simulink library "xblocks_library_pfbs"  (Simulink 7.6)
settings: Solver=ode45  SolverMode=SingleTasking  StartTime=0.0  StopTime=10.0  RelTol=1e-3
libraries: xbsIndex_r4 x369, monroe_library x47
(part 2 of 7)

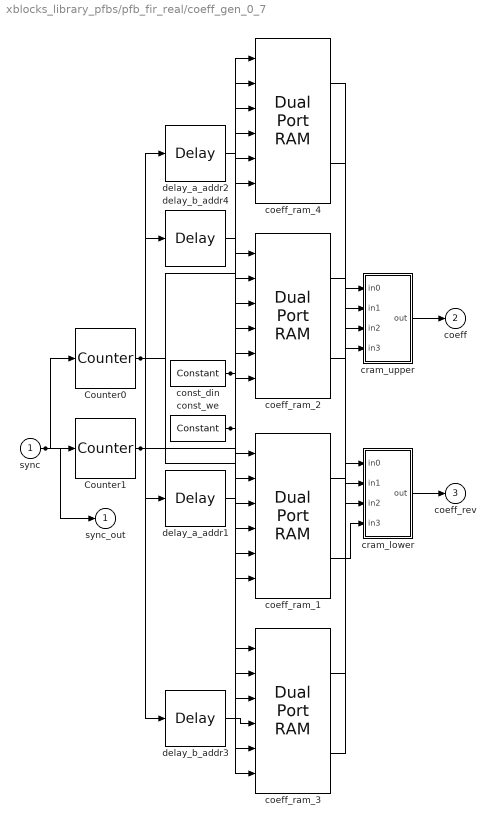
== system xblocks_library_pfbs/pfb_fir_real/coeff_gen_0_7 ==
  sync : Inport
  Counter0 : xbsIndex_r4/Counter  cnt_type=Free Running  cnt_to=Inf  operation=Up  start_count=8  cnt_by_val=1  arith_type=Unsigned  n_bits=11  bin_pt=0  load_pin=off  rst=on  en=off  explicit_period=on  period=1  dbl_ovrd=off  use_behavioral_HDL=off  implementation=Fabric  block_type=counter
  Counter1 : xbsIndex_r4/Counter  cnt_type=Free Running  cnt_to=Inf  operation=Down  start_count=2039  cnt_by_val=1  arith_type=Unsigned  n_bits=11  bin_pt=0  load_pin=off  rst=on  en=off  explicit_period=on  period=1  dbl_ovrd=off  use_behavioral_HDL=off  implementation=Fabric  block_type=counter
  coeff_ram_1 : xbsIndex_r4/Dual Port RAM  depth=2048  initVector=[-1.22072174986674e-006 -2.07573634838521e-005 -4.03037029782619e-005 -5.98598996980381e-005 -7.94261132606548e-005 -9.90025034347064e-005 -0.000118589230138382 -0.00013818645343805 -0.000157794333546782 -0.000177413030822893 -0.000197042705768457 -0.000216683519027889 -0.000236335631386401 -0.00025599920376858 -0.000275674397236896 -0.000295361372990216 -0.000315060292362373 -0.00033477131682061 -0.000354494607964151 -0.000374230327522695 -0.000393978637354936 -0.000413739699447062 -0.000433513675911303 -0.000453300728984377 -0.000473101021026037 -0.000492914714517562 -0.000512741972060248 -0.000532582956373951 -0.00055243783029552 -0.000572306756777332 -0.000592189898885775 -0.000612087419799743 -0.000631999482809111 -0.00065192625131327 -0.000671867888819539 -0.000691824558941702 -0.000711796425398473 -0.000731783652011965 -0.000751786402706218 -0.0007718048415056 -0.000791839132533333 -0.000811889440009951 -0.00083195592825177 -0.000852038761669347 -0.000872138104765997 -0.000892254122136178 -0.000912386978464012 -0.000932536838521728 -0.000952703867168116 -0.000972888229347025 -0.000993090090085754 -0.00101330961449355 -0.00103354696776005 -0.00105380231515375 -0.00107407582202039 -0.00109436765378152 -0.00111467797593281 -0.0011350069540426 -0.00115535475375027 -0.00117572154076472 -0.00119610748086284 -0.00121651273988784 -0.00123693748374781 -0.00125738187841406 -0.00127784608991962 -0.0012983302843576 -0.0013188346278797 -0.00133935928669459 -0.00135990442706632 -0.00138047021531278 -0.00140105681780409 -0.00142166440096108 -0.00144229313125365 -0.00146294317519918 -0.001483614699361 -0.00150430787034677 -0.0015250228548069 -0.00154575981943296 -0.00156651893095611 -0.00158730035614545 -0.00160810426180649 -0.00162893081477952 -0.00164978018193805 -0.00167065253018717 -0.00169154802646197 -0.00171246683772591 -0.00173340913096929 -0.00175437507320756 -0.00177536483147979 -0.00179637857284702 -0.00181741646439064 -0.00183847867321083 -0.00185956536642487 -0.00188067671116564 -0.00190181287457992 -0.00192297402382678 -0.001944160326076 -0.00196537194850642 -0.00198660905830434 -0.00200787182266191 -0.00202916040877547 -0.00205047498384395 -0.00207181571506724 -0.00209318276964456 -0.00211457631477287 -0.00213599651764518 -0.00215744354544895 -0.00217891756536446 -0.00220041874456319 -0.00222194725020613 -0.00224350324944225 -0.00226508690940674 -0.00228669839721945 -0.00230833787998322 -0.00233000552478227 -0.00235170149868053 -0.00237342596871999 -0.0023951791019191 -0.00241696106527107 -0.00243877202574225 -0.00246061215027048 -0.00248248160576349 -0.00250438055909712 -0.00252630917711381 -0.00254826762662086 -0.0025702560743888 -0.00259227468714977 -0.00261432363159582 -0.00263640307437723 -0.00265851318210093 -0.00268065412132879 -0.00270282605857593 -0.00272502916030915 -0.0027472635929452 -0.00276952952284908 -0.00279182711633249 -0.00281415653965204 -0.0028365179590077 -0.00285891154054103 -0.00288133745033356 -0.00290379585440513 -0.00292628691871219 -0.00294881080914613 -0.00297136769153166 -0.00299395773162504 -0.0030165810951125 -0.00303923794760849 -0.00306192845465405 -0.00308465278171512 -0.00310741109418087 -0.00313020355736198 -0.003153030336489 -0.00317589159671066 -0.00319878750309216 -0.00322171822061356 -0.00324468391416799 -0.00326768474856006 -0.0032907208885041 -0.00331379249862253 -0.00333689974344414 -0.00336004278740241 -0.00338322179483382 -0.00340643692997616 -0.00342968835696683 -0.00345297623984116 -0.00347630074253073 -0.00349966202886164 -0.00352306026255283 -0.00354649560721441 -0.00356996822634591 -0.00359347828333467 -0.00361702594145403 -0.00364061136386173 -0.00366423471359816 -0.00368789615358466 -0.00371159584662182 -0.00373533395538786 -0.00375911064243679 -0.00378292607019678 -0.00380678040096848 -0.00383067379692324 -0.00385460642010154 -0.00387857843241112 -0.00390258999562537 -0.00392664127138162 -0.00395073242117942 -0.00397486360637879 -0.00399903498819863 ...(+37251 chars)]  distributed_mem=Block RAM  init_a=0  init_b=0  rst_a=off  rst_b=off  en_a=off  en_b=off  latency=2  write_mode_A=No Read On Write  write_mode_B=No Read On Write  dbl_ovrd=off  optimize=Area  use_rpm=on  block_type=dpram
  coeff_ram_2 : xbsIndex_r4/Dual Port RAM  depth=2048  initVector=[1.64803315783465e-005 0.000280485521810809 0.000545093027402636 0.00081030310745065 0.00107611601953105 0.00134253201969671 0.00160955136247522 0.00187717430086683 0.00214540108634176 0.00241423196883855 0.00268366719676137 0.00295370701697797 0.00322435167481777 0.00349560141406919 0.00376745647697767 0.00403991710424374 0.00431298353502034 0.00458665600691093 0.00486093475596747 0.00513582001668779 0.00541131202201398 0.00568741100332972 0.00596411719045836 0.00624143081166097 0.00651935209363378 0.0067978812615062 0.00707701853883898 0.00735676414762159 0.00763711830827029 0.00791808123962629 0.00819965315895307 0.00848183428193485 0.008764624822674 0.00904802499368911 0.00933203500591316 0.00961665506869093 0.00990188538977718 0.0101877261753347 0.010474177629932 0.010761239956541 0.0110489133565358 0.0113371980296895 0.0116260941741733 0.0119156019865533 0.0122057216617891 0.012496453393232 0.0127877973726222 0.0130797537900872 0.0133723228341399 0.0136655046916763 0.0139592995479734 0.0142537075866877 0.0145487289898524 0.0148443639378762 0.0151406126095406 0.0154374751819983 0.0157349518307712 0.0160330427297483 0.0163317480511835 0.0166310679656943 0.0169310026422588 0.0172315522482147 0.017532716949257 0.0178344969094354 0.0181368922911536 0.0184399032551663 0.0187435299605775 0.019047772564839 0.0193526312237478 0.0196581060914447 0.0199641973204122 0.0202709050614723 0.020578229463785 0.0208861706748463 0.021194728840486 0.0215039041048662 0.0218136966104791 0.0221241064981451 0.0224351339070113 0.0227467789745491 0.0230590418365527 0.0233719226271371 0.0236854214787361 0.0239995385221007 0.0243142738862971 0.0246296276987047 0.0249456000850147 0.0252621911692277 0.0255794010736522 0.0258972299189029 0.0262156778238985 0.0265347449058598 0.0268544312803088 0.0271747370610656 0.0274956623602476 0.0278172072882672 0.02813937195383 0.0284621564639336 0.0287855609238648 0.0291095854371986 0.0294342301057965 0.029759495029804 0.0300853803076495 0.0304118860360423 0.0307390123099709 0.0310667592227011 0.0313951268657746 0.0317241153290068 0.0320537247004856 0.0323839550665691 0.0327148065118842 0.0330462791193253 0.0333783729700515 0.0337110881434859 0.0340444247173137 0.03437838276748 0.0347129623681887 0.0350481635919005 0.0353839865093313 0.0357204311894507 0.0360574976994799 0.0363951861048906 0.0367334964694028 0.0370724288549838 0.0374119833218455 0.0377521599284443 0.0380929587314779 0.0384343797858845 0.0387764231448415 0.0391190888597629 0.0394623769802986 0.0398062875543322 0.0401508206279795 0.0404959762455876 0.0408417544497322 0.0411881552812166 0.0415351787790705 0.0418828249805475 0.0422310939211244 0.0425799856344993 0.0429295001525897 0.0432796375055317 0.0436303977216779 0.0439817808275958 0.0443337868480668 0.0446864158060843 0.045039667722852 0.0453935426177829 0.0457480405084974 0.0461031614108218 0.0464589053387873 0.0468152723046275 0.0471722623187784 0.0475298753898752 0.0478881115247521 0.0482469707284406 0.0486064530041675 0.0489665583533539 0.0493272867756139 0.0496886382687526 0.0500506128287651 0.0504132104498352 0.0507764311243331 0.0511402748428151 0.0515047415940217 0.0518698313648757 0.0522355441404818 0.0526018799041244 0.0529688386372664 0.0533364203195482 0.0537046249287857 0.0540734524409694 0.0544429028302629 0.0548129760690015 0.0551836721276905 0.0555549909750048 0.0559269325777866 0.0562994969010446 0.0566726839079523 0.0570464935598469 0.0574209258162282 0.0577959806347566 0.0581716579712526 0.058547957779695 0.0589248800122198 0.0593024246191185 0.0596805915488377 0.0600593807479768 0.0604387921612875 0.0608188257316721 0.0611994814001824 0.0615807591060186 0.0619626587865276 0.062345180377202 0.0627283238116794 0.0631120890217402 0.063496475937307 0.0638814844864433 0.064267114595352 0.0646533661883749 0.0650402391879906 0.0654277335148137 0.065815849087594 0.0662045858232146 0.0665939436366913 0.0669839224411714 0.067374522147932 0.0677657426663793 0.0681575839040475 ...(+32994 chars)]  distributed_mem=Block RAM  init_a=0  init_b=0  rst_a=off  rst_b=off  en_a=off  en_b=off  latency=2  write_mode_A=No Read On Write  write_mode_B=No Read On Write  dbl_ovrd=off  optimize=Area  use_rpm=on  block_type=dpram
  coeff_ram_3 : xbsIndex_r4/Dual Port RAM  depth=2048  initVector=[0.999999997939492 0.999999404513317 0.999997756108682 0.999995052729556 0.999991294382447 0.999986481076405 0.99998061282302 0.999973689636421 0.999965711533277 0.999956678532798 0.999946590656734 0.999935447929374 0.999923250377545 0.999909998030619 0.999895690920501 0.999880329081641 0.999863912551025 0.999846441368179 0.999827915575169 0.9998083352166 0.999787700339613 0.999766010993892 0.999743267231656 0.999719469107664 0.999694616679213 0.999668710006138 0.999641749150811 0.999613734178142 0.999584665155579 0.999554542153107 0.999523365243246 0.999491134501054 0.999457850004128 0.999423511832596 0.999388120069126 0.999351674798921 0.999314176109716 0.999275624091786 0.999236018837938 0.999195360443513 0.999153649006388 0.999110884626972 0.999067067408209 0.999022197455575 0.99897627487708 0.998929299783265 0.998881272287205 0.998832192504505 0.998782060553301 0.998730876554262 0.998678640630587 0.998625352908004 0.998571013514771 0.998515622581677 0.998459180242038 0.998401686631699 0.998343141889033 0.998283546154941 0.998222899572851 0.998161202288718 0.998098454451022 0.998034656210769 0.997969807721491 0.997903909139244 0.997836960622608 0.997768962332688 0.997699914433111 0.997629817090025 0.997558670472104 0.99748647475054 0.997413230099047 0.997338936693861 0.997263594713734 0.997187204339941 0.997109765756274 0.997031279149043 0.996951744707075 0.996871162621715 0.996789533086822 0.996706856298774 0.99662313245646 0.996538361761285 0.996452544417169 0.996365680630542 0.996277770610348 0.996188814568043 0.996098812717592 0.996007765275471 0.995915672460666 0.995822534494672 0.99572835160149 0.99563312400763 0.995536851942108 0.995439535636445 0.995341175324669 0.99524177124331 0.995141323631404 0.995039832730486 0.994937298784596 0.994833722040274 0.994729102746561 0.994623441154996 0.994516737519617 0.994408992096962 0.994300205146064 0.99419037692845 0.994079507708148 0.993967597751674 0.993854647328043 0.993740656708758 0.993625626167818 0.99350955598171 0.993392446429412 0.99327429779239 0.993155110354601 0.993034884402484 0.99291362022497 0.992791318113473 0.992667978361889 0.9925436012666 0.992418187126472 0.992291736242848 0.992164248919555 0.992035725462898 0.99190616618166 0.991775571387104 0.991643941392966 0.99151127651546 0.991377577073273 0.991242843387566 0.991107075781971 0.990970274582594 0.990832440118009 0.990693572719259 0.990553672719856 0.990412740455777 0.990270776265469 0.990127780489838 0.989983753472259 0.989838695558565 0.989692607097053 0.989545488438481 0.989397339936062 0.989248161945471 0.989097954824838 0.988946718934749 0.988794454638243 0.988641162300815 0.988486842290409 0.988331494977421 0.988175120734697 0.988017719937532 0.987859292963666 0.987699840193286 0.987539362009025 0.987377858795956 0.987215330941599 0.98705177883591 0.986887202871287 0.986721603442567 0.986554980947023 0.986387335784363 0.986218668356731 0.986048979068703 0.985878268327288 0.985706536541923 0.985533784124477 0.985360011489246 0.985185219052951 0.985009407234739 0.98483257645618 0.984654727141269 0.984475859716419 0.984295974610463 0.984115072254653 0.983933153082657 0.983750217530559 0.983566266036857 0.98338129904246 0.983195316990689 0.983008320327275 0.982820309500356 0.982631284960478 0.982441247160591 0.98225019655605 0.98205813360461 0.981865058766429 0.981670972504062 0.981475875282465 0.981279767568986 0.981082649833371 0.980884522547757 0.980685386186674 0.980485241227041 0.980284088148167 0.980081927431746 0.979878759561857 0.979674585024966 0.979469404309918 0.97926321790794 0.979056026312637 0.978847830019992 0.978638629528364 0.978428425338485 0.978217217953461 0.978005007878768 0.977791795622251 0.977577581694123 0.977362366606961 0.97714615087571 0.976928935017675 0.97671071955252 0.976491505002273 0.976271291891314 0.976050080746383 0.975827872096571 0.975604666473324 0.975380464410436 0.975155266444051 0.974929073112661 0.9747018849571 0.97447370252055 0.974244526348531 ...(+32991 chars)]  distributed_mem=Block RAM  init_a=0  init_b=0  rst_a=off  rst_b=off  en_a=off  en_b=off  latency=2  write_mode_A=No Read On Write  write_mode_B=No Read On Write  dbl_ovrd=off  optimize=Area  use_rpm=on  block_type=dpram
  coeff_ram_4 : xbsIndex_r4/Dual Port RAM  depth=2048  initVector=[-1.64779798652932e-005 -0.000279805876911002 -0.000542532014217755 -0.000804656655620616 -0.00106618006646648 -0.00132710251361138 -0.00158742426541843 -0.00184714559175581 -0.00210626676399397 -0.00236478805500397 -0.00262270973915464 -0.0028800320923106 -0.00313675539183012 -0.00339287991656244 -0.00364840594684571 -0.00390333376450485 -0.00415766365284889 -0.00441139589666884 -0.0046645307822356 -0.00491706859729718 -0.0051690096310769 -0.00542035417427064 -0.00567110251904467 -0.00592125495903356 -0.00617081178933743 -0.00641977330651982 -0.00666813980860556 -0.006915911595078 -0.00716308896687689 -0.00740967222639621 -0.00765566167748135 -0.0079010576254273 -0.00814586037697581 -0.0083900702403132 -0.00863368752506823 -0.00887671254230929 -0.00911914560454224 -0.00936098702570823 -0.00960223712118088 -0.00984289620776415 -0.0100829646036901 -0.0103224426286159 -0.0105613306036224 -0.0107996288512106 -0.0110373376953001 -0.0112744574612263 -0.0115109884757381 -0.0117469310669953 -0.0119822855645665 -0.0122170522994264 -0.0124512316039533 -0.0126848238119272 -0.0129178292585265 -0.0131502482803265 -0.013382081215296 -0.0136133284027958 -0.0138439901835755 -0.0140740668997713 -0.0143035588949036 -0.0145324665138748 -0.014760790102966 -0.0149885300098353 -0.0152156865835152 -0.0154422601744097 -0.0156682511342925 -0.0158936598163037 -0.0161184865749479 -0.0163427317660917 -0.0165663957469608 -0.0167894788761377 -0.0170119815135596 -0.0172339040205152 -0.0174552467596424 -0.0176760100949264 -0.017896194391696 -0.0181158000166224 -0.0183348273377156 -0.0185532767243224 -0.0187711485471239 -0.0189884431781327 -0.0192051609906904 -0.0194213023594655 -0.0196368676604501 -0.0198518572709579 -0.0200662715696215 -0.02028011093639 -0.0204933757525261 -0.0207060664006037 -0.0209181832645053 -0.0211297267294199 -0.0213406971818396 -0.0215510950095574 -0.021760920601665 -0.0219701743485495 -0.0221788566418916 -0.0223869678746622 -0.0225945084411204 -0.0228014787368109 -0.0230078791585608 -0.0232137101044777 -0.0234189719739467 -0.0236236651676281 -0.0238277900874542 -0.0240313471366275 -0.0242343367196175 -0.024436759242158 -0.0246386151112452 -0.0248399047351341 -0.0250406285233368 -0.0252407868866192 -0.0254403802369984 -0.0256394089877407 -0.0258378735533583 -0.0260357743496066 -0.0262331117934824 -0.0264298863032203 -0.0266260982982904 -0.0268217481993957 -0.0270168364284696 -0.0272113634086729 -0.0274053295643913 -0.0275987353212325 -0.0277915811060242 -0.0279838673468106 -0.0281755944728502 -0.028366762914613 -0.0285573731037779 -0.0287474254732299 -0.0289369204570574 -0.0291258584905497 -0.0293142400101941 -0.0295020654536733 -0.0296893352598626 -0.0298760498688275 -0.0300622097218205 -0.0302478152612788 -0.0304328669308217 -0.0306173651752471 -0.0308013104405299 -0.0309847031738184 -0.0311675438234319 -0.0313498328388582 -0.0315315706707505 -0.0317127577709246 -0.0318933945923569 -0.0320734815891808 -0.0322530192166844 -0.0324320079313076 -0.0326104481906397 -0.0327883404534162 -0.0329656851795162 -0.03314248282996 -0.0333187338669057 -0.0334944387536472 -0.0336695979546105 -0.0338442119353522 -0.0340182811625555 -0.034191806104028 -0.0343647872286992 -0.0345372250066172 -0.0347091199089462 -0.0348804724079639 -0.0350512829770582 -0.0352215520907249 -0.0353912802245649 -0.0355604678552809 -0.0357291154606754 -0.0358972235196473 -0.0360647925121894 -0.0362318229193854 -0.0363983152234075 -0.036564269907513 -0.0367296874560422 -0.0368945683544149 -0.0370589130891282 -0.0372227221477533 -0.0373859960189329 -0.0375487351923784 -0.0377109401588668 -0.0378726114102382 -0.038033749439393 -0.0381943547402887 -0.0383544278079377 -0.0385139691384038 -0.0386729792288 -0.0388314585772849 -0.0389894076830611 -0.0391468270463708 -0.0393037171684944 -0.0394600785517467 -0.0396159116994746 -0.0397712171160541 -0.0399259953068873 -0.0400802467783997 -0.0402339720380375 -0.0403871715942645 -0.0405398459565594 -0.0406919956354128 ...(+37233 chars)]  distributed_mem=Block RAM  init_a=0  init_b=0  rst_a=off  rst_b=off  en_a=off  en_b=off  latency=2  write_mode_A=No Read On Write  write_mode_B=No Read On Write  dbl_ovrd=off  optimize=Area  use_rpm=on  block_type=dpram
  const_din : xbsIndex_r4/Constant  const=0  gui_display_data_type=Fixed-point  arith_type=Signed (2's comp)  n_bits=18  bin_pt=17  preci_type=Single  exp_width=8  frac_width=24  explicit_period=on  period=1  equ=P=C  opselect=C  inp2=PCIN>>17  opr=+  inp1=P  carry=CIN  dbl_ovrd=off  block_type=constant
  const_we : xbsIndex_r4/Constant  const=0  gui_display_data_type=Fixed-point  arith_type=Boolean  n_bits=16  bin_pt=14  preci_type=Single  exp_width=8  frac_width=24  explicit_period=on  period=1  equ=P=C  opselect=C  inp2=PCIN>>17  opr=+  inp1=P  carry=CIN  dbl_ovrd=off  block_type=constant
  cram_lower : Subsystem
  cram_upper : Subsystem
  delay_a_addr1 : xbsIndex_r4/Delay  rst=off  infoeditControl=Selection of Reset will increase slice count due to use of real FFs and instead of SRLs  en=off  latency=2  dbl_ovrd=off  reg_retiming=off  block_type=delay
  delay_a_addr2 : xbsIndex_r4/Delay  rst=off  infoeditControl=Selection of Reset will increase slice count due to use of real FFs and instead of SRLs  en=off  latency=1  dbl_ovrd=off  reg_retiming=off  block_type=delay
  delay_b_addr3 : xbsIndex_r4/Delay  rst=off  infoeditControl=Selection of Reset will increase slice count due to use of real FFs and instead of SRLs  en=off  latency=1  dbl_ovrd=off  reg_retiming=off  block_type=delay
  delay_b_addr4 : xbsIndex_r4/Delay  rst=off  infoeditControl=Selection of Reset will increase slice count due to use of real FFs and instead of SRLs  en=off  latency=2  dbl_ovrd=off  reg_retiming=off  block_type=delay
  sync_out : Outport
  coeff : Outport  Port=2
  coeff_rev : Outport  Port=3
  wires:
  sync/1 -> Counter1/1, Counter0/1, sync_out/1
  Counter0/1 -> coeff_ram_4/1, coeff_ram_3/1, delay_a_addr2/1, delay_a_addr1/1
  const_din/1 -> coeff_ram_4/5, coeff_ram_4/2, coeff_ram_3/5, coeff_ram_3/2, coeff_ram_2/5, coeff_ram_2/2, coeff_ram_1/5, coeff_ram_1/2
  const_we/1 -> coeff_ram_4/6, coeff_ram_4/3, coeff_ram_3/6, coeff_ram_3/3, coeff_ram_2/6, coeff_ram_2/3, coeff_ram_1/6, coeff_ram_1/3
  Counter1/1 -> delay_b_addr4/1, delay_b_addr3/1, coeff_ram_2/4, coeff_ram_1/4
  cram_lower/1(out) -> coeff_rev/1
  cram_upper/1(out) -> coeff/1
  coeff_ram_1/2 -> cram_lower/4(in3)
  coeff_ram_2/2 -> cram_lower/3(in2)
  coeff_ram_3/2 -> cram_lower/2(in1)
  coeff_ram_4/2 -> cram_lower/1(in0)
  coeff_ram_4/1 -> cram_upper/4(in3)
  coeff_ram_3/1 -> cram_upper/3(in2)
  coeff_ram_2/1 -> cram_upper/2(in1)
  coeff_ram_1/1 -> cram_upper/1(in0)
  delay_b_addr4/1 -> coeff_ram_4/4
  delay_b_addr3/1 -> coeff_ram_3/4
  delay_a_addr2/1 -> coeff_ram_2/1
  delay_a_addr1/1 -> coeff_ram_1/1
